simulink library "TM_Standalone_Library"  (Simulink 7.8)
settings: Solver=ode45  StartTime=0.0  StopTime=10.0  RelTol=1e-3
settings Model: Creator=vpadmaj  LastModifiedBy=vpadmaj

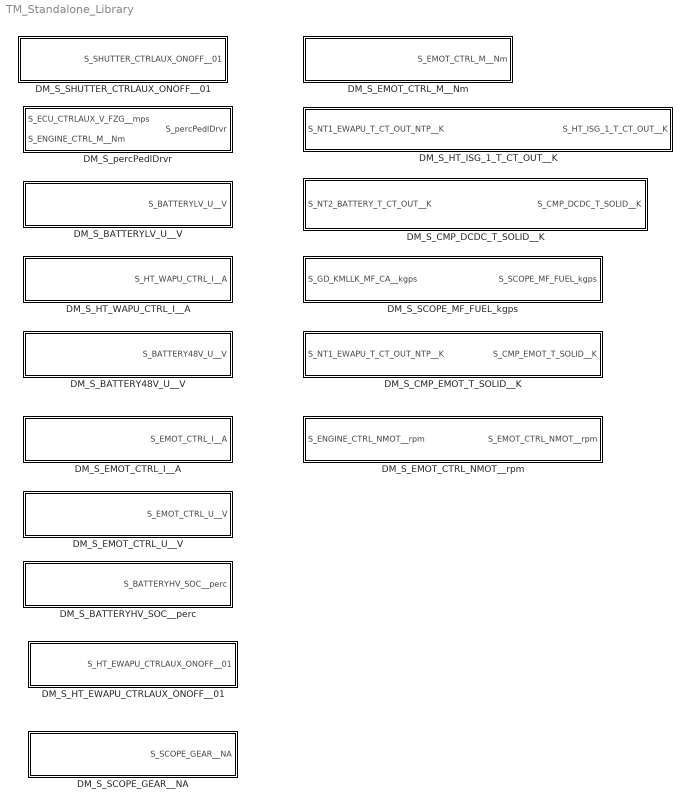
== system TM_Standalone_Library ==
  DM_S_BATTERY48V_U__V : Subsystem
  DM_S_BATTERYHV_SOC__perc : Subsystem
  DM_S_BATTERYLV_U__V : Subsystem
  DM_S_CMP_DCDC_T_SOLID__K : Subsystem
  DM_S_CMP_EMOT_T_SOLID__K : Subsystem
  DM_S_EMOT_CTRL_I__A : Subsystem
  DM_S_EMOT_CTRL_M__Nm : Subsystem
  DM_S_EMOT_CTRL_NMOT__rpm : Subsystem
  DM_S_EMOT_CTRL_U__V : Subsystem
  DM_S_HT_EWAPU_CTRLAUX_ONOFF__01 : Subsystem
  DM_S_HT_ISG_1_T_CT_OUT__K : Subsystem
  DM_S_HT_WAPU_CTRL_I__A : Subsystem
  DM_S_SCOPE_GEAR__NA : Subsystem
  DM_S_SCOPE_MF_FUEL_kgps : Subsystem
  DM_S_SHUTTER_CTRLAUX_ONOFF__01 : Subsystem
  DM_S_percPedlDrvr : Subsystem

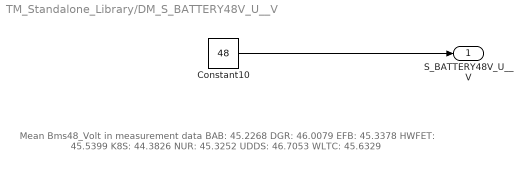
== system TM_Standalone_Library/DM_S_BATTERY48V_U__V ==
  note: Mean Bms48_Volt in measurement data
      | BAB: 45.2268
      | DGR: 46.0079
      | EFB: 45.3378
      | HWFET: 45.5399
      | K8S:  44.3826
      | NUR: 45.3252
      | UDDS: 46.7053
      | WLTC: 45.6329
  Constant10 : Constant  Value=48
  S_BATTERY48V_U__V : Outport
  wires:
  Constant10/1 -> S_BATTERY48V_U__V/1

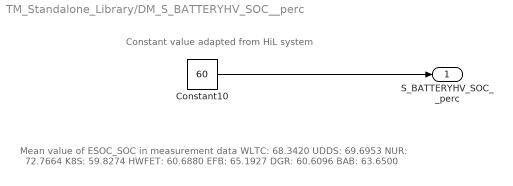
== system TM_Standalone_Library/DM_S_BATTERYHV_SOC__perc ==
  note: Constant value adapted from HiL system
  note: Mean value of ESOC_SOC in measurement data
      | WLTC: 68.3420
      | UDDS: 69.6953
      | NUR: 72.7664
      | K8S: 59.8274
      | HWFET: 60.6880
      | EFB: 65.1927
      | DGR: 60.6096
      | BAB: 63.6500
  Constant10 : Constant  Value=60
  S_BATTERYHV_SOC__perc : Outport
  wires:
  Constant10/1 -> S_BATTERYHV_SOC__perc/1

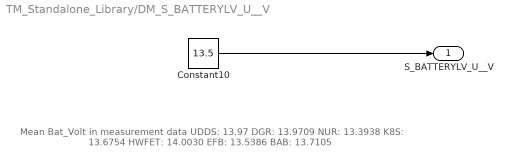
== system TM_Standalone_Library/DM_S_BATTERYLV_U__V ==
  note: Mean Bat_Volt in measurement data
      | UDDS: 13.97
      | DGR: 13.9709
      | NUR: 13.3938
      | K8S: 13.6754
      | HWFET: 14.0030
      | EFB: 13.5386
      | BAB: 13.7105
  Constant10 : Constant  Value=13.5
  S_BATTERYLV_U__V : Outport
  wires:
  Constant10/1 -> S_BATTERYLV_U__V/1

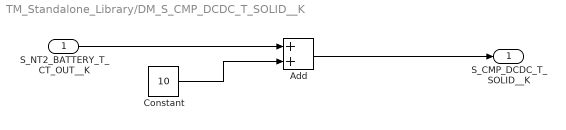
== system TM_Standalone_Library/DM_S_CMP_DCDC_T_SOLID__K ==
  S_NT2_BATTERY_T_CT_OUT__K : Inport
  Add : Sum
  Constant : Constant  Value=10
  S_CMP_DCDC_T_SOLID__K : Outport
  wires:
  S_NT2_BATTERY_T_CT_OUT__K/1 -> Add/1
  Add/1 -> S_CMP_DCDC_T_SOLID__K/1
  Constant/1 -> Add/2

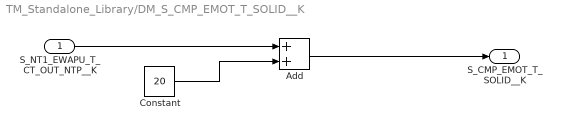
== system TM_Standalone_Library/DM_S_CMP_EMOT_T_SOLID__K ==
  S_NT1_EWAPU_T_CT_OUT_NTP__K : Inport
  Add : Sum
  Constant : Constant  Value=20
  S_CMP_EMOT_T_SOLID__K : Outport
  wires:
  Constant/1 -> Add/2
  Add/1 -> S_CMP_EMOT_T_SOLID__K/1
  S_NT1_EWAPU_T_CT_OUT_NTP__K/1 -> Add/1

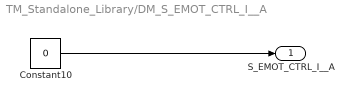
== system TM_Standalone_Library/DM_S_EMOT_CTRL_I__A ==
  Constant10 : Constant  Value=0
  S_EMOT_CTRL_I__A : Outport
  wires:
  Constant10/1 -> S_EMOT_CTRL_I__A/1

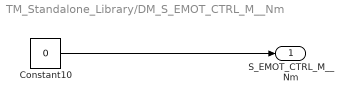
== system TM_Standalone_Library/DM_S_EMOT_CTRL_M__Nm ==
  Constant10 : Constant  Value=0
  S_EMOT_CTRL_M__Nm : Outport
  wires:
  Constant10/1 -> S_EMOT_CTRL_M__Nm/1

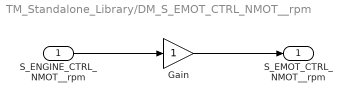
== system TM_Standalone_Library/DM_S_EMOT_CTRL_NMOT__rpm ==
  S_ENGINE_CTRL_NMOT__rpm : Inport
  Gain : Gain
  S_EMOT_CTRL_NMOT__rpm : Outport
  wires:
  S_ENGINE_CTRL_NMOT__rpm/1 -> Gain/1
  Gain/1 -> S_EMOT_CTRL_NMOT__rpm/1

== system TM_Standalone_Library/DM_S_EMOT_CTRL_U__V ==
  note: Mean values of EM2_Volt in measurement data
      | BAB: 45.2693
      | DGR: 45.3021
      | EFB: 45.1758
      | HWFET: 45.3485
      | K8S: 44.3883
      | NUR: 45.5211
      | UDDS: 46.0209
  Constant10 : Constant  Value=45.3
  S_EMOT_CTRL_U__V : Outport
  wires:
  Constant10/1 -> S_EMOT_CTRL_U__V/1

== system TM_Standalone_Library/DM_S_HT_EWAPU_CTRLAUX_ONOFF__01 ==
  note: This is a waterpump on request from HVAC
  Constant10 : Constant  Value=0
  S_HT_EWAPU_CTRLAUX_ONOFF__01 : Outport
  wires:
  Constant10/1 -> S_HT_EWAPU_CTRLAUX_ONOFF__01/1

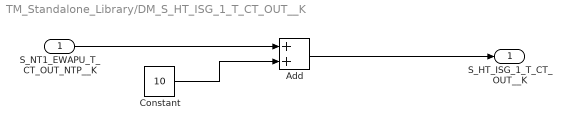
== system TM_Standalone_Library/DM_S_HT_ISG_1_T_CT_OUT__K ==
  S_NT1_EWAPU_T_CT_OUT_NTP__K : Inport
  Add : Sum
  Constant : Constant  Value=10
  S_HT_ISG_1_T_CT_OUT__K : Outport
  wires:
  S_NT1_EWAPU_T_CT_OUT_NTP__K/1 -> Add/1
  Add/1 -> S_HT_ISG_1_T_CT_OUT__K/1
  Constant/1 -> Add/2

== system TM_Standalone_Library/DM_S_HT_WAPU_CTRL_I__A ==
  Constant10 : Constant  Value=0
  S_HT_WAPU_CTRL_I__A : Outport
  wires:
  Constant10/1 -> S_HT_WAPU_CTRL_I__A/1

== system TM_Standalone_Library/DM_S_SCOPE_GEAR__NA ==
  Constant10 : Constant  Value=0
  S_SCOPE_GEAR__NA : Outport
  wires:
  Constant10/1 -> S_SCOPE_GEAR__NA/1

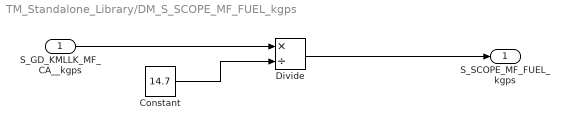
== system TM_Standalone_Library/DM_S_SCOPE_MF_FUEL_kgps ==
  S_GD_KMLLK_MF_CA__kgps : Inport
  Constant : Constant  Value=14.7
  Divide : Product  Inputs=*/
  S_SCOPE_MF_FUEL_kgps : Outport
  wires:
  Constant/1 -> Divide/2
  Divide/1 -> S_SCOPE_MF_FUEL_kgps/1
  S_GD_KMLLK_MF_CA__kgps/1 -> Divide/1

== system TM_Standalone_Library/DM_S_SHUTTER_CTRLAUX_ONOFF__01 ==
  note: Shutter On request from HVAC
  Constant10 : Constant  Value=0
  S_SHUTTER_CTRLAUX_ONOFF__01 : Outport
  wires:
  Constant10/1 -> S_SHUTTER_CTRLAUX_ONOFF__01/1

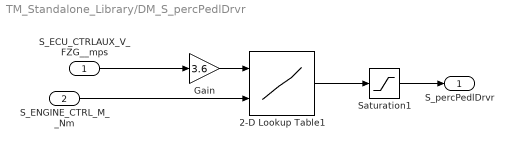
== system TM_Standalone_Library/DM_S_percPedlDrvr ==
  S_ECU_CTRLAUX_V_FZG__mps : Inport
  S_ENGINE_CTRL_M__Nm : Inport  Port=2
  2-D Lookup Table1 : Lookup_n-D  BreakpointsForDimension1=[-100:50:600]  BreakpointsForDimension2=[0:20:260]'  Table=|  RndMeth=Simplest  InputSameDT=on
      | [0.136532010091195	1.06506062587129	1.44105702629421	0.497003826898518	18.3719280240781	32.0089779306973	-0.0613502373842147	3.26166386833152	-3.28520194826759	6.75863200136261	6.75863200136261	6.75863200136261	6.75863200136261	6.75863200136261
      | 0.136532010091195	1.06506062587129	1.44105702629421	0.497003826898518	18.3719280240781	32.0089779306973	-0.0613502373842147	3.26166386833152	-3.28520194826759	6.75863200136261	6.75863200136261	6.75863200136261	6.75863200136261	6.75863200136261
      | 0.136532010091195	1.06506062587129	1.44105702629421	0.497003826898518	18.3719280240781	32.0089779306973	-0.0613502373842147	3.26166386833152	-3.28520194826759	6.75863200136261	6.75863200136261	6.75863200136261	6.75863200136261	6.75863200136261
      | 0.136532010091195	1.06506062587129	1.44105702629421	-0.469882423455665	30.7243640280007	24.8771488515614	-4.10649310352249	1.85467747357131	-3.28520194826759	20.4713045262861	20.4713045262861	20.4713045262861	20.4713045262861	20.4713045262861
      | 0.136532010091195	6.36000676257024	6.60812276192469	17.3712238699306	12.9664425243199	30.3453211546949	11.5999607559656	28.2705711888003	9.71764561714246	23.8032095643684	23.8032095643684	23.8032095643684	23.8032095643684	23.8032095643684
      | 5.97552415540025	16.0397603748792	14.4928936340754	16.3818458257828	23.1702627158638	14.0340040944166	21.3750045960033	22.3349355970766	15.3407694863040	23.9623288075284	23.9623288075284	23.9623288075284	23.9623288075284	23.9623288075284
      | 28.7163602285886	28.7163602285886	18.6836922546518	24.3314780941815	46.4113702232814	34.3986291035619	67.1306127746408	28.3606357699889	26.0980124720935	93.6458107274116	93.6458107274116	93.6458107274116	93.6458107274116	93.6458107274116
      | 26.9085185569282	26.9085185569282	29.0293476319464	32.5226164850991	69.9591368560043	32.3574448335667	43.2514178057416	33.7429131981850	30.3516397899794	92.1310652029881	92.1310652029881	92.1310652029881	92.1310652029881	92.1310652029881
      | 42.4676757275990	42.4676757275990	43.9695243397579	36.9900628656814	70.2496086671159	39.7878436421410	67.2988431849512	37.4819835817244	36.9555651868164	80.7281561802862	80.7281561802862	80.7281561802862	80.7281561802862	80.7281561802862
      | 42.9984466530504	42.9984466530504	45.0260100317765	46.2912070421018	59.6185057139539	44.6173947167594	40.6630774815570	70.6709967016388	79.7187003917478	99.9798540792469	99.9798540792469	99.9798540792469	99.9798540792469	99.9798540792469
      | 46.6376556854565	46.6376556854565	46.8987648017386	50.2803621332203	49.4369853576106	49.0271319385651	46.5778540939131	75.0240067124223	85.5914611360396	98.7656826773592	98.7656826773592	98.7656826773592	98.7656826773592	98.7656826773592
      | 52.8899714101104	52.8899714101104	54.4113820918227	53.1440284028890	43.9549451984172	49.9887762969358	51.9227670881972	84.2352123450504	82.0362980633087	96.7605363919919	96.7605363919919	96.7605363919919	96.7605363919919	96.7605363919919
      | 77.3212781599724	77.3212781599724	77.3212781599724	56.0042830665705	100.252993682630	100.000000000000	97.0424345524934	100	90.7556503501609	98.6120896030947	98.6120896030947	98.6120896030947	98.6120896030947	98.6120896030947
      | 100.830667809427	100.830667809427	100.830667809427	100.830667809427	100.830667809427	100.830667809427	100.830667809427	100.830667809427	100.830667809427	100.830667809427	100.830667809427	100.830667809427	100.830667809427	100.830667809427
      | 100.830667809427	100.830667809427	100.830667809427	100.830667809427	100.830667809427	100.830667809427	100.830667809427	100.830667809427	100.830667809427	100.830667809427	100.830667809427	100.830667809427	100.830667809427	100.830667809427
      | ]
  Gain : Gain  Gain=3.6
  Saturation1 : Saturate  UpperLimit=100  LowerLimit=0
  S_percPedlDrvr : Outport
  wires:
  2-D Lookup Table1/1 -> Saturation1/1
  S_ENGINE_CTRL_M__Nm/1 -> 2-D Lookup Table1/2
  S_ECU_CTRLAUX_V_FZG__mps/1 -> Gain/1
  Saturation1/1 -> S_percPedlDrvr/1
  Gain/1 -> 2-D Lookup Table1/1
